simulink model "teta2puntos "  (R2016a)
settings: Solver=FixedStepAuto  StartTime=0.0  StopTime=100  FixedStep=0.001  RelTol=1e-3
settings Model: Creator=usuario17  LastModifiedBy=User

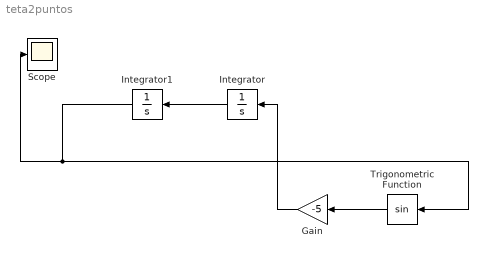
== system teta2puntos  ==
  Gain : Gain  Gain=-5
  Integrator : Integrator  InitialCondition=pi/2
  Integrator1 : Integrator  InitialCondition=pi/2
  Scope : Scope
  Trigonometric Function : Trigonometry
  wires:
  Integrator/1 -> Integrator1/1
  Integrator1/1 -> Scope/1, Trigonometric Function/1
  Trigonometric Function/1 -> Gain/1
  Gain/1 -> Integrator/1
